simulink model "flowSpeedCalculation_th"  (R2018b)
settings: Solver=FixedStepAuto  StartTime=0.0  StopTime=duration_s  FixedStep=1  RelTol=1e-3
undefined symbols (not defined in the file or in its folder): env, nodeDrag, nodeDragForce_ul, nodePosToLinkPos, nodePosToLinkPos_ul, variableFlow, variableFlow_ul
libraries: dspmtrx3 x4, Dynamic_2D_Lookup_Table x3, variableFlowProfileCalculation_ul x3, simulink x1
settings Model: Creator=James Reed  LastModifiedBy=James Reed

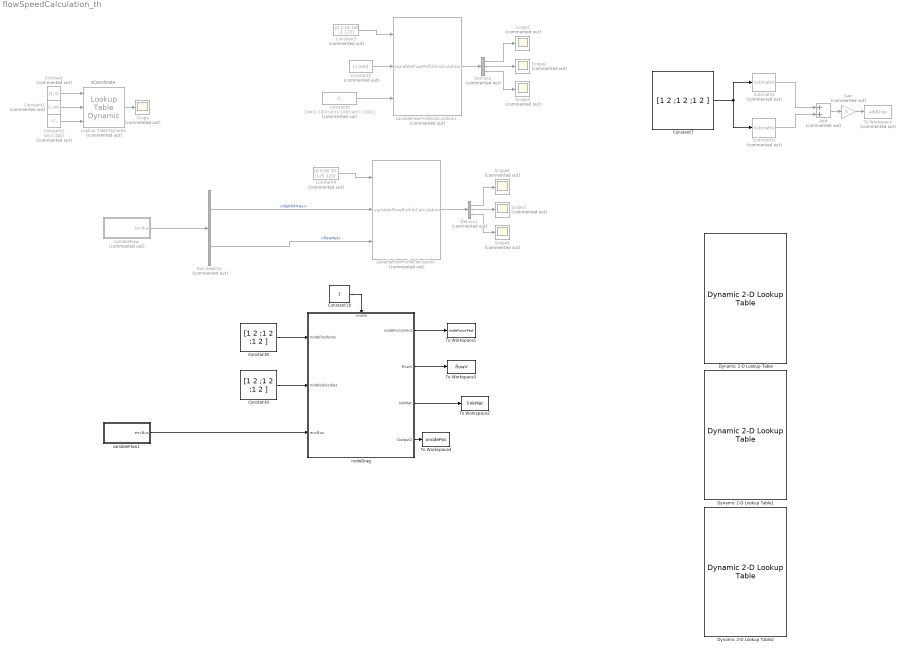
== system flowSpeedCalculation_th ==
  note: xCoordinate
  Add : Sum  Commented=on
  Bus Selector : BusSelector  Commented=on  OutputSignals=depthArray,flowMat
  Constant : Constant  Commented=on  Value=[1;3]
  Constant1 : Constant  Commented=on  Value=[1:100]
  Constant10 : Constant
  Constant2 : Constant  Commented=on  Value=sin(1:100)
  Constant3 : Constant  Commented=on  Value=[0 2;50 100 ;1 125]
  Constant4 : Constant  Commented=on  Value=[0 0;50 50 ;125 125]
  Constant5 : Constant  Commented=on  Value=[1:100]
  Constant6 : Constant  Commented=on  Value=[sin(1:100);sin(1:100);sin(1:100);]
  Constant7 : Constant  Value=[1 2 ;1 2 ;1 2 ]
  Constant8 : Constant  Value=[1 2 ;1 2 ;1 2 ]
  Constant9 : Constant  Value=[1 2 ;1 2 ;1 2 ]
  Demux1 : Demux  Commented=on  Outputs=3
  Demux2 : Demux  Commented=on  Outputs=3
  Dynamic 2-D Lookup Table : Dynamic_2D_Lookup_Table/Dynamic 2-D Lookup Table
  Dynamic 2-D Lookup Table1 : Dynamic_2D_Lookup_Table/Dynamic 2-D Lookup Table
  Dynamic 2-D Lookup Table2 : Dynamic_2D_Lookup_Table/Dynamic 2-D Lookup Table
  Gain : Gain  Commented=on  Gain=.5
  Lookup Table Dynamic : simulink/Lookup Tables/Lookup Table Dynamic  Commented=on  LookUpMeth=Interpolation-Use End Values  OutDataType=fixdt('double')  OutScaling=[]  OutputDataTypeScalingMode=Specify via dialog  OutDataTypeStr=double  DoSatur=off
      settings: SourceProductName=Simulink
  Scope{,1..3,6..8} (7 alike) : Scope  Commented=on
  Submatrix : dspmtrx3/Submatrix  Commented=on  RowSpan=All rows  RowStartMode=First  RowStartIndex=1  RowEndMode=Last  RowEndIndex=1  ColSpan=Range of columns  ColStartMode=First  ColStartIndex=1  ColEndMode=Offset from last  ColEndIndex=1
  Submatrix1 : dspmtrx3/Submatrix  Commented=on  RowSpan=All rows  RowStartMode=First  RowStartIndex=1  RowEndMode=Last  RowEndIndex=1  ColSpan=Range of columns  ColStartMode=Index  ColStartIndex=2  ColEndMode=Last  ColEndIndex=1
  To Workspace : ToWorkspace  Commented=on  VariableName=addDisp  SaveFormat=Timeseries  SampleTime=-1
  To Workspace1 : ToWorkspace  VariableName=nodeForceTest  SaveFormat=Timeseries  SampleTime=-1
  To Workspace2 : ToWorkspace  VariableName=linkMat  SaveFormat=Timeseries  SampleTime=-1
  To Workspace3 : ToWorkspace  VariableName=flowV  SaveFormat=Timeseries  SampleTime=-1
  To Workspace4 : ToWorkspace  VariableName=onodePos  SaveFormat=Timeseries  SampleTime=-1
  nodeDrag : Subsystem  AncestorBlock=nodeDragForce_ul/nodeDrag  mask{flowDensity=1000, thrDiam=.0144, dragCoeff=2}
      mask prompts: flowDensity "Flow Density"; thrDiam "Tether Diameter"; dragCoeff "Drag Coefficient"
  variableFlow : Subsystem  Commented=on  AncestorBlock=variableFlow_ul/variableFlow  VariantControl=VSS_environment_constantUniformFlow
  variableFlow1 : Subsystem  AncestorBlock=variableFlow_ul/variableFlow  VariantControl=VSS_environment_constantUniformFlow
  variableFlowProfileCalculation : variableFlowProfileCalculation_ul/variableFlowProfileCalculation  Commented=on  SystemSampleTime=-1
  variableFlowProfileCalculation1 : variableFlowProfileCalculation_ul/variableFlowProfileCalculation  Commented=on  SystemSampleTime=-1
  wires:
  Constant4/1 -> variableFlowProfileCalculation/1
  variableFlow/1(envBus) -> Bus Selector/1
  Demux1/3 -> Scope8/1
  Demux1/2 -> Scope7/1
  Demux1/1 -> Scope6/1
  variableFlowProfileCalculation/1 -> Demux1/1
  Constant/1 -> Lookup Table Dynamic/1
  Lookup Table Dynamic/1 -> Scope/1
  Bus Selector/1 -> variableFlowProfileCalculation/2  "<depthArray>"
  Bus Selector/2 -> variableFlowProfileCalculation/3  "<flowMat>"
  Constant1/1 -> Lookup Table Dynamic/2
  Constant2/1 -> Lookup Table Dynamic/3
  Demux2/2 -> Scope2/1
  Demux2/3 -> Scope3/1
  Demux2/1 -> Scope1/1
  Constant3/1 -> variableFlowProfileCalculation1/1
  variableFlowProfileCalculation1/1 -> Demux2/1
  Constant5/1 -> variableFlowProfileCalculation1/2
  Constant6/1 -> variableFlowProfileCalculation1/3
  Add/1 -> Gain/1
  Constant7/1 -> Submatrix1/1, Submatrix/1
  Submatrix1/1 -> Add/2
  Submatrix/1 -> Add/1
  Gain/1 -> To Workspace/1
  variableFlow1/1(envBus) -> nodeDrag/3("envBus ")
  nodeDrag/1(nodeForceVecs) -> To Workspace1/1
  Constant8/1 -> nodeDrag/1(nodePositions)
  Constant9/1 -> nodeDrag/2(nodeVelocities)
  nodeDrag/2("flowV ") -> To Workspace3/1
  nodeDrag/3("linkMat ") -> To Workspace2/1
  nodeDrag/4(Output2) -> To Workspace4/1
  Constant10/1 -> nodeDrag/Enable

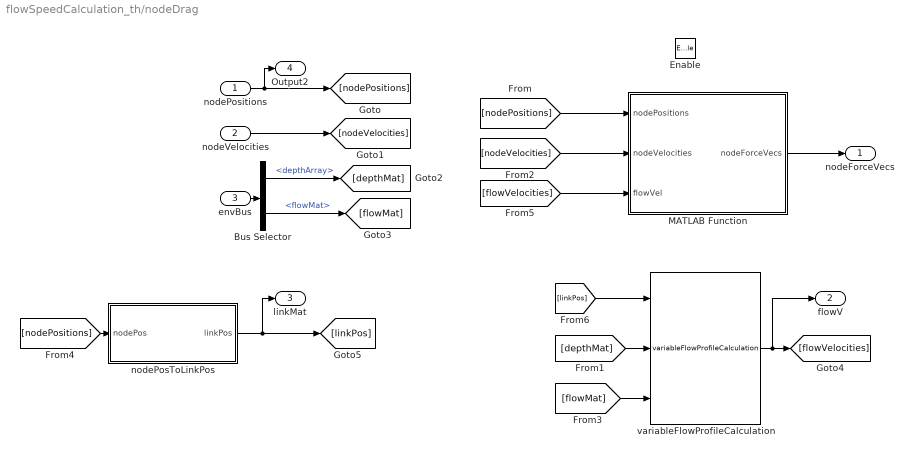
== system flowSpeedCalculation_th/nodeDrag ==
  nodePositions : Inport
  nodeVelocities : Inport  Port=2
  "envBus " : Inport  Port=3  OutDataTypeStr=Bus: envBus
  Enable : EnablePort
  Bus Selector : BusSelector  OutputSignals=depthArray,flowMat
  MATLAB Function : MATLAB Function  TreatAsAtomicUnit=on
  nodePosToLinkPos : Subsystem  AncestorBlock=nodePosToLinkPos_ul/nodePosToLinkPos
  variableFlowProfileCalculation : variableFlowProfileCalculation_ul/variableFlowProfileCalculation  SystemSampleTime=-1
  nodeForceVecs : Outport
  "flowV " : Outport  Port=2
  "linkMat " : Outport  Port=3
  Output2 : Outport  Port=4
  wires:
  [nodePositions] -> nodePosToLinkPos/1("nodePos ")
  [linkPos] -> variableFlowProfileCalculation/1
  nodePosToLinkPos/1("linkPos ") -> "linkMat "/1, [linkPos]
  variableFlowProfileCalculation/1 -> "flowV "/1, [flowVelocities]
  [flowMat] -> variableFlowProfileCalculation/3
  [depthMat] -> variableFlowProfileCalculation/2
  Bus Selector/2 -> [flowMat]  "<flowMat>"
  Bus Selector/1 -> [depthMat]  "<depthArray>"
  "envBus "/1 -> Bus Selector/1
  nodeVelocities/1 -> [nodeVelocities]
  [nodePositions] -> MATLAB Function/1(nodePositions)
  MATLAB Function/1(nodeForceVecs) -> nodeForceVecs/1
  [flowVelocities] -> MATLAB Function/3(flowVel)
  [nodeVelocities] -> MATLAB Function/2(nodeVelocities)
  nodePositions/1 -> Output2/1, [nodePositions]

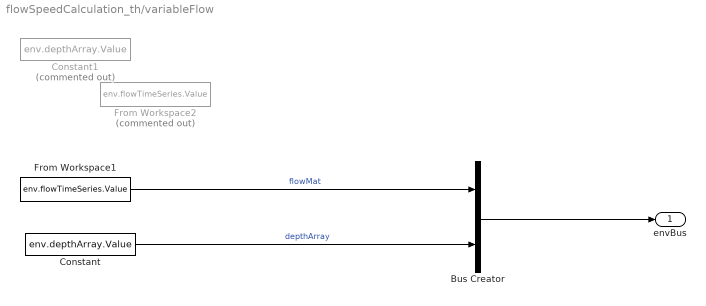
== system flowSpeedCalculation_th/variableFlow ==
  Bus Creator : BusCreator  Inputs=2  OutDataTypeStr=Bus: envBus
  Constant : Constant  Value=env.depthArray.Value
  Constant1 : Constant  Commented=on  Value=env.depthArray.Value
  From Workspace1 : FromWorkspace  VariableName=env.flowTimeSeries.Value  SampleTime=0
  From Workspace2 : FromWorkspace  Commented=on  VariableName=env.flowTimeSeries.Value  SampleTime=0
  envBus : Outport  OutDataTypeStr=Bus: envBus
  wires:
  Constant/1 -> Bus Creator/2  "depthArray"
  From Workspace1/1 -> Bus Creator/1  "flowMat"
  Bus Creator/1 -> envBus/1

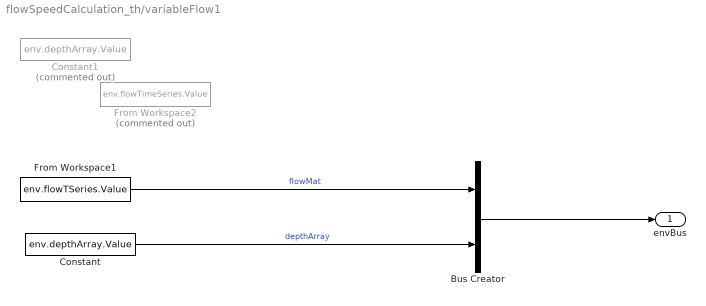
== system flowSpeedCalculation_th/variableFlow1 ==
  Bus Creator : BusCreator  Inputs=2  OutDataTypeStr=Bus: envBus
  Constant : Constant  Value=env.depthArray.Value
  Constant1 : Constant  Commented=on  Value=env.depthArray.Value
  From Workspace1 : FromWorkspace  VariableName=env.flowTSeries.Value  SampleTime=0
  From Workspace2 : FromWorkspace  Commented=on  VariableName=env.flowTimeSeries.Value  SampleTime=0
  envBus : Outport  OutDataTypeStr=Bus: envBus
  wires:
  Constant/1 -> Bus Creator/2  "depthArray"
  From Workspace1/1 -> Bus Creator/1  "flowMat"
  Bus Creator/1 -> envBus/1

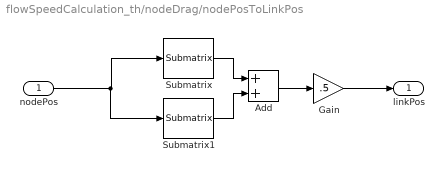
== system flowSpeedCalculation_th/nodeDrag/nodePosToLinkPos ==
  "nodePos " : Inport
  Add : Sum
  Gain : Gain  Gain=.5
  Submatrix : dspmtrx3/Submatrix  RowSpan=All rows  RowStartMode=First  RowStartIndex=1  RowEndMode=Last  RowEndIndex=1  ColSpan=Range of columns  ColStartMode=First  ColStartIndex=1  ColEndMode=Offset from last  ColEndIndex=1
  Submatrix1 : dspmtrx3/Submatrix  RowSpan=All rows  RowStartMode=First  RowStartIndex=1  RowEndMode=Last  RowEndIndex=1  ColSpan=Range of columns  ColStartMode=Index  ColStartIndex=2  ColEndMode=Last  ColEndIndex=1
  "linkPos " : Outport
  wires:
  Submatrix1/1 -> Add/2
  Submatrix/1 -> Add/1
  Add/1 -> Gain/1
  Gain/1 -> "linkPos "/1
  "nodePos "/1 -> Submatrix/1, Submatrix1/1

== matlab function flowSpeedCalculation_th/nodeDrag/MATLAB Function ==
  data: nodePositions input; nodeForceVecs output; nodeVelocities input; thrDiam parameter; flowDensity parameter; flowVel input; dragCoeff parameter
function nodeForceVecs = fcn(nodePositions,nodeVelocities,thrDiam, flowDensity, flowVel,dragCoeff)
% In the notation here, N is the number of nodes, therefore you have N-1
% links between the nodes.

% Velocity and center of links 3xN-1
linkVelocities = (nodeVelocities(:,1:end-1) + nodeVelocities(:,2:end))/2;

% Apparent flow at center of links 3xN-1
linkAppFlow = flowVel - linkVelocities; %repmat(flowVel(:),[1 size(linkVelocities,2)]) - linkVelocities;
% linkAppFlow(3,:) = 0; % Origional model zeroed z component

% Link center apparent flow magnitude 3xN-1
linkAppFlowMag = sqrt(sum(linkAppFlow.^2)); % Sum over columns

% Normalize columns to get unit vector 3xN-1
dragDirUnitVec = linkAppFlow./repmat(linkAppFlowMag,[3 1]);

% If linkAppFlowMag is zero, dragDirUnitVec will have nans, patch to fix
% that with zeros
% dragDirUnitVec(:,linkAppFlowMag==0) = zeros(3,numel(linkAppFlowMag==0));

% Dynamic pressures at link centers 1xN-1
dynPress = 0.5*flowDensity*linkAppFlowMag.^2;

% Link lengths, diff over columns 1xN-1
linkLengths = sqrt(sum(diff(nodePositions,1,2).^2));

% Unit vectors in the direction of the link 3xN-1
linkUnitVecs = diff(nodePositions,1,2)./repmat(linkLengths,[3 1]);

% Projected areas of each link
projArea = thrDiam*linkLengths.*sqrt(sum(cross(linkUnitVecs,dragDirUnitVec).^2,1));

% Drag force on links
linkForceVecs = repmat(dragCoeff*dynPress.*projArea,[3 1]).*dragDirUnitVec;

% Drag force on nodes
nodeForceVecs = [linkForceVecs(:,1) (linkForceVecs(:,1:end-1)+linkForceVecs(:,2:end)) linkForceVecs(:,end)]/2;

end
